simulink model "race"  (R2018a)
settings: Solver=VariableStepAuto  StartTime=0.0  StopTime=300  FixedStep=0.01  RelTol=1e-3
values from neighbouring files (symbols this model uses):
  gates = sim_gates(:,:,1)    [eval_sim.m]    (also in initialize_race_realtime.m = [dist,0,height,deg2rad(110); initialize_race_realtime_backup_cubic.m = [dist,0,height,deg2rad(110); plot_sim.m)
  splines = zeros(3,4,size(gates,1))    [initialize_race_no_realtime.m]    (also in show_splines.m)
undefined symbols (not defined in the file or in its folder): fspecial, gray, Rec, SDTV
libraries: visiontextngfix x2, visionanalysis x1, visiontransforms x1, visionconversions x1, vrlib x1
settings Model: Creator=vinni  LastModifiedBy=vinni

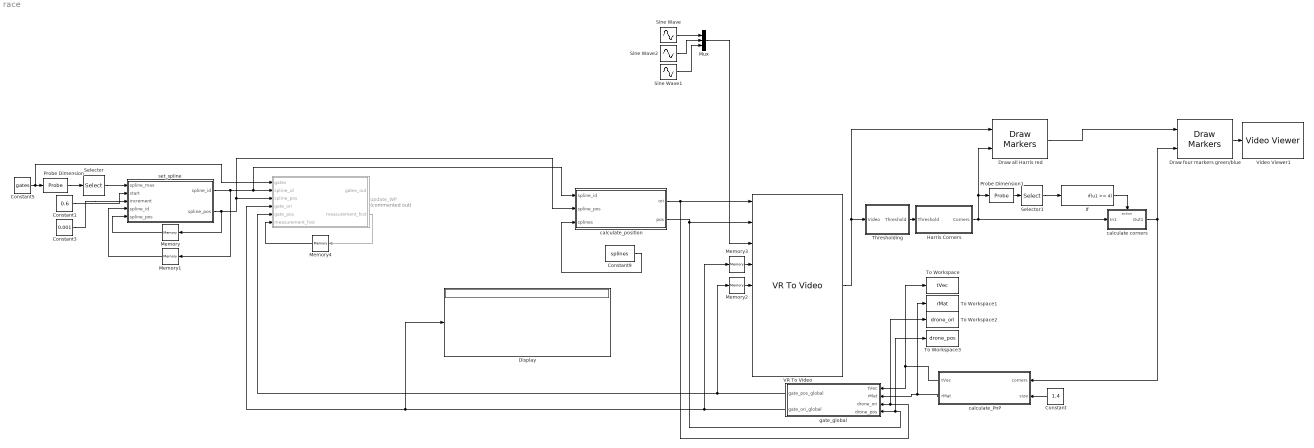
== system race ==
  Constant : Constant  Value=1.4
  Constant1 : Constant  Value=0.6
  Constant3 : Constant  Value=0.001
  Constant5 : Constant  Value=gates
  Constant9 : Constant  Value=splines
  Display : Display
  Draw all Harris red : visiontextngfix/Draw Markers  shape=Circle  size=3  fill=on  fillClrSource=Specify via dialog  display=User-specified value  intensity=200  color=[255 0 0]  opacity=1  viewport=Entire image  antialiasing=off  inType=Obsolete  imagePorts=One multidimensional signal  prodOutputMode=Binary point scaling  prodOutputWordLength=32  prodOutputFracLength=14  memoryMode=Specify word length  memoryWordLength=16  memoryFracLength=14  roundingMode=Floor  overflowMode=off
      settings: SourceProductName=Computer Vision System Toolbox  SourceProductBaseCode=VP
  Draw four markers green/blue : visiontextngfix/Draw Markers  shape=Circle  size=3  fill=on  fillClrSource=Specify via dialog  display=User-specified value  intensity=200  color=[0 255 0; 0 0 255;0 0 255; 0 255 0]  opacity=1  viewport=Entire image  antialiasing=off  inType=Obsolete  imagePorts=One multidimensional signal  prodOutputMode=Binary point scaling  prodOutputWordLength=32  prodOutputFracLength=14  memoryMode=Specify word length  memoryWordLength=16  memoryFracLength=14  roundingMode=Floor  overflowMode=off
      settings: SourceProductName=Computer Vision System Toolbox  SourceProductBaseCode=VP
  Harris Corners : Subsystem
  If : If  IfExpression=u1 >= 4  ShowElse=off
  Memory{,1..4} (5 alike) : Memory
  Mux : Mux  Inputs=3
  Probe Dimension : Probe  ProbeWidth=off  ProbeSampleTime=off  ProbeComplexSignal=off  ProbeSignalDimensions=on
  Probe Dimension1 : Probe  ProbeWidth=off  ProbeSampleTime=off  ProbeComplexSignal=off  ProbeSignalDimensions=on
  Selector : Selector  IndexOptions=Index vector (dialog)  Indices=1  OutputSizes=1
  Selector1 : Selector  IndexOptions=Index vector (dialog)  Indices=1  OutputSizes=1
  Sine Wave : Sin  Amplitude=0.0  Bias=3  Frequency=0.4  SampleTime=0
  Sine Wave1 : Sin  Amplitude=0.0  Bias=2  Frequency=0.4  SampleTime=0
  Sine Wave2 : Sin  Amplitude=0.0  Frequency=0.4  SampleTime=0
  Thresholding : Subsystem
  To Workspace : ToWorkspace  VariableName=tVec  SaveFormat=Timeseries  SampleTime=-1
  To Workspace1 : ToWorkspace  VariableName=rMat  SaveFormat=Timeseries  SampleTime=-1
  To Workspace2 : ToWorkspace  VariableName=drone_ori  SaveFormat=Timeseries  SampleTime=-1
  To Workspace3 : ToWorkspace  VariableName=drone_pos  SaveFormat=Timeseries  SampleTime=-1
  VR To Video : vrlib/VR To Video  InstantiateOnLoad=on  SampleTime=0.1  ViewEnable=on  RemoteChange=off  RemoteView=off  FieldsWritten=drone.orientation.4.1.1.double#drone.position.3.1.1.double#G1.translation.3.1.1.double#current_gate_red.rotation.4.1.1.double#current_gate_red.translation.3.1.1.double#current_gate_yellow.rotation.4.1.1.double#current_gate_yellow.translation.3.1.1.double#current_gate_green.rotation.4.1.1.double#current_gate_green.translation.3.1.1.double  WorldFileName=race_course.wrl  AutoView=off  VideoDimensions=1*[200 320]  AllowVariableSize=off  FigureProperties="{'Position', 'Name', 'Viewpoint', 'CameraBound', 'CameraDirection', 'CameraPosition', 'CameraUpVector', 'ZoomFactor', 'Antialiasing', 'Headlight', 'Lighting', 'NavPanel', 'Sound', 'StatusBar', 'Stereo3D', 'Stereo3DCameraOffset', 'Stereo3DHIT', 'ToolBar', 'Textures', 'Transparency', 'Triad', 'Wireframe', 'NavZones', 'NavMode', 'NavSpeed', 'CaptureFileFormat', 'CaptureFileName', 'Record2DCompressMethod', 'Record2DCompressQuality', 'Record2D', 'Record2DFileName', 'Record2DFPS'; [3.5500000000000000e+02   6.0000000000000000e+01   3.2000000000000000e+02   2.0000000000000000e+02], '', '_untitled_1', 'on', [0.0000000000000000e+00   0.0000000000000000e+00  -1.0000000000000000e+00], [0.0000000000000000e+00   0.0000000000000000e+00   0.0000000000000000e+00], [0.0000000000000000e+00   1.0000000000000000e+00   0.0000000000000000e+00], [1.0000000000000000e+00], 'on', 'on', 'on', 'none', 'on', 'off', 'off', [1.0000000149011612e-01], [0.0000000000000000e+00], 'off', 'on', 'on', 'none', 'off', 'off', 'fly', 'normal', 'tif', '%f_anim_%n.tif', 'auto', [7.5000000000000000e+01], 'off', '***video***', 'auto'}"
      settings: SourceProductName=Simulink 3D Animation  SourceProductBaseCode=VR
  Video Viewer1 : VideoViewer  colormapValue=gray(256)  FigPos=[66 898 1535 821]
  calculate corners : Subsystem  TreatAsAtomicUnit=on
  calculate_PnP : MATLAB Function  TreatAsAtomicUnit=on
  calculate_position : MATLAB Function  TreatAsAtomicUnit=on
  gate_global : MATLAB Function  TreatAsAtomicUnit=on
  set_spline : MATLAB Function  TreatAsAtomicUnit=on
  update_WP : MATLAB Function  Commented=on  TreatAsAtomicUnit=on
  wires:
  Sine Wave2/1 -> Mux/2
  Sine Wave/1 -> Mux/1
  Sine Wave1/1 -> Mux/3
  VR To Video/1 -> Draw all Harris red/1, Thresholding/1("Video ")
  Probe Dimension/1 -> Selector/1
  Selector/1 -> set_spline/1(spline_max)
  Constant5/1 -> update_WP/1(gates), Probe Dimension/1
  Memory1/1 -> set_spline/4("spline_id ")
  Memory/1 -> set_spline/5("spline_pos ")
  Constant9/1 -> calculate_position/3(splines)
  calculate_position/1(ori) -> To Workspace2/1, gate_global/3(drone_ori), VR To Video/1
  Draw all Harris red/1 -> Draw four markers green/blue/1
  Thresholding/1(Threshold) -> Harris Corners/1(Threshold)
  Harris Corners/1(Corners) -> Draw all Harris red/2, Probe Dimension1/1, calculate corners/1(In1)
  Constant/1 -> calculate_PnP/2(size)
  Probe Dimension1/1 -> Selector1/1
  Selector1/1 -> If/1
  calculate corners/1(Out1) -> calculate_PnP/1(corners), Draw four markers green/blue/2
  calculate_position/2(pos) -> To Workspace3/1, gate_global/4(drone_pos), VR To Video/2
  calculate_PnP/1(tVec) -> gate_global/1(tVec), To Workspace/1
  If/1 -> calculate corners/Action
  Draw four markers green/blue/1 -> Video Viewer1/1
  Constant3/1 -> set_spline/3(increment)
  calculate_PnP/2(rMat) -> gate_global/2(rMat), To Workspace1/1
  gate_global/1(gate_pos_global) -> update_WP/5(gate_pos), Memory2/1
  Constant1/1 -> set_spline/2(start)
  gate_global/2(gate_ori_global) -> Display/1, update_WP/4(gate_ori), Memory3/1
  Mux/1 -> VR To Video/3
  Memory3/1 -> VR To Video/4
  Memory2/1 -> VR To Video/5
  update_WP/2(measurement_hist) -> Memory4/1
  Memory4/1 -> update_WP/6("measurement_hist ")
  set_spline/1(spline_id) -> Memory1/1, calculate_position/1(spline_id), update_WP/2(spline_id)
  set_spline/2(spline_pos) -> Memory/1, calculate_position/2(spline_pos), update_WP/3(spline_pos)

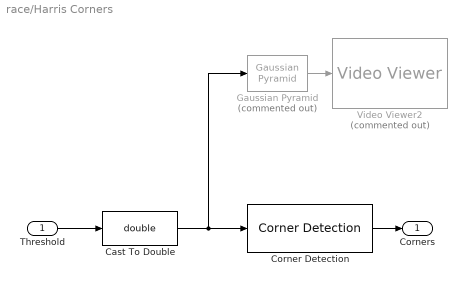
== system race/Harris Corners ==
  Threshold : Inport
  Cast To Double : DataTypeConversion  OutDataTypeStr=double
  Corner Detection : visionanalysis/Corner Detection  method=Harris corner detection (Harris & Stephens)  factor=0.01  filter=fspecial('gaussian', [1 9], 3)  thrInten=0.1  thrAngle=157.5  output=Obsolete9b  outputInUse=Corner location  maxNum=5  thrMetric=0.01  neighborSize=[25 25]  isOutVarDim=on  accumMode=Binary point scaling  accumWordLength=32  accumFracLength=0  prodOutputMode=Binary point scaling  prodOutputWordLength=32  prodOutputFracLength=0  memoryMode=Binary point scaling  memoryWordLength=32  memoryFracLength=0  firstCoeffMode=Specify word length  firstCoeffWordLength=16  firstCoeffFracLength=17  roundingMode=Floor  overflowMode=off
      settings: SourceProductName=Computer Vision System Toolbox  SourceProductBaseCode=VP
  Gaussian Pyramid : visiontransforms/Gaussian Pyramid  Commented=on  operation=Expand  level=1  source=Specify via dialog  a=0.375  coef=fspecial('gaussian', [1 9], 3)  hiddenCoef=fspecial('gaussian', [1 9], 3)  firstCoeffMode=Specify word length  firstCoeffWordLength=16  firstCoeffFracLength=17  outputMode=Binary point scaling  outputWordLength=32  outputFracLength=10  prodOutputMode=Binary point scaling  prodOutputWordLength=32  prodOutputFracLength=10  roundingMode=Floor  overflowMode=off
      settings: SourceProductName=Computer Vision System Toolbox  SourceProductBaseCode=VP
  Video Viewer2 : VideoViewer  Commented=on  colormapValue=gray(256)  FigPos=[66 898 768 793]
  Corners : Outport
  wires:
  Threshold/1 -> Cast To Double/1
  Cast To Double/1 -> Gaussian Pyramid/1, Corner Detection/1
  Gaussian Pyramid/1 -> Video Viewer2/1
  Corner Detection/1 -> Corners/1

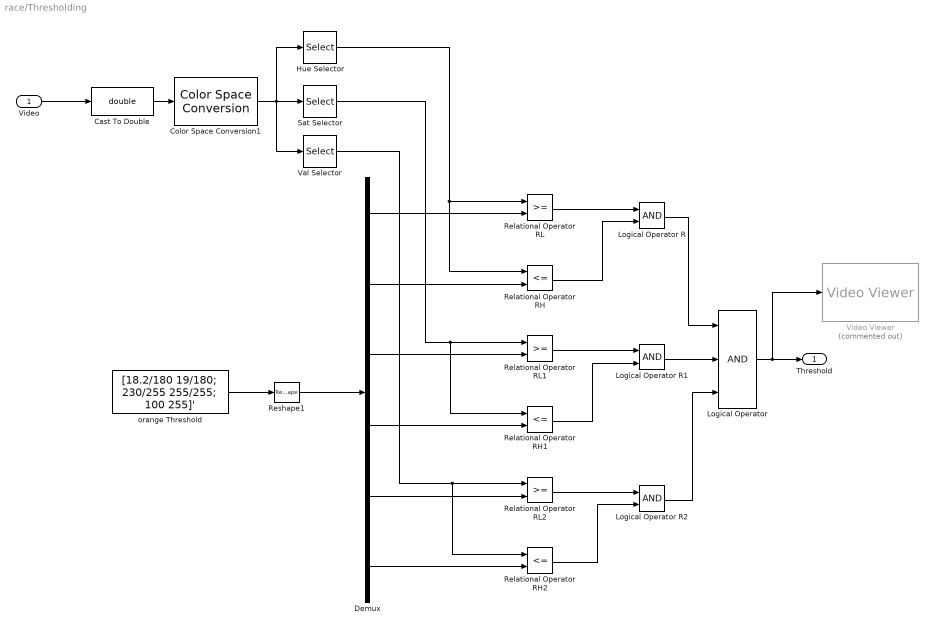
== system race/Thresholding ==
  "Video " : Inport
  Cast To Double : DataTypeConversion  OutDataTypeStr=double
  Color Space Conversion1 : visionconversions/Color Space  Conversion  conversion=Obsolete  conversionActive=R'G'B' to HSV  wp_str=D65  rec=Rec. 601 (SDTV)  sys=1125/60/2:1  imagePorts=One multidimensional signal
      settings: SourceProductName=Computer Vision System Toolbox
  Demux : Demux  Outputs=6
  Hue Selector : Selector  NumberOfDimensions=3  InputPortWidth=3  IndexOptions=Select all,Select all,Index vector (dialog)  Indices=[1 3],1,1  OutputSizes=1,1,1
  Logical Operator : Logic  Inputs=3  AllPortsSameDT=off  OutDataTypeStr=boolean
  Logical Operator R : Logic  AllPortsSameDT=off  OutDataTypeStr=boolean
  Logical Operator R1 : Logic  AllPortsSameDT=off  OutDataTypeStr=boolean
  Logical Operator R2 : Logic  AllPortsSameDT=off  OutDataTypeStr=boolean
  Relational Operator RH : RelationalOperator  Operator=<=  OutDataTypeStr=boolean  RndMeth=Nearest
  Relational Operator RH1 : RelationalOperator  Operator=<=  OutDataTypeStr=boolean  RndMeth=Nearest
  Relational Operator RH2 : RelationalOperator  Operator=<=  OutDataTypeStr=boolean  RndMeth=Nearest
  Relational Operator RL : RelationalOperator  OutDataTypeStr=boolean  RndMeth=Nearest
  Relational Operator RL1 : RelationalOperator  OutDataTypeStr=boolean  RndMeth=Nearest
  Relational Operator RL2 : RelationalOperator  OutDataTypeStr=boolean  RndMeth=Nearest
  Reshape1 : Reshape
  Sat Selector : Selector  NumberOfDimensions=3  InputPortWidth=3  IndexOptions=Select all,Select all,Index vector (dialog)  Indices=[1 3],1,2  OutputSizes=1,1,1
  Val Selector : Selector  NumberOfDimensions=3  InputPortWidth=3  IndexOptions=Select all,Select all,Index vector (dialog)  Indices=[1 3],1,3  OutputSizes=1,1,1
  Video Viewer : VideoViewer  Commented=on  colormapValue=gray(256)  FigPos=[66 898 1535 821]
  orange Threshold : Constant  Value=[18.2/180 19/180; 230/255 255/255; 100 255]'  OutDataTypeStr=double
  Threshold : Outport
  wires:
  Color Space Conversion1/1 -> Val Selector/1, Sat Selector/1, Hue Selector/1
  Demux/6 -> Relational Operator RH2/2
  Val Selector/1 -> Relational Operator RH2/1, Relational Operator RL2/1
  Demux/3 -> Relational Operator RL1/2
  Relational Operator RL/1 -> Logical Operator R/1
  Demux/2 -> Relational Operator RH/2
  orange Threshold/1 -> Reshape1/1
  Cast To Double/1 -> Color Space Conversion1/1
  Demux/5 -> Relational Operator RL2/2
  Hue Selector/1 -> Relational Operator RH/1, Relational Operator RL/1
  Logical Operator R/1 -> Logical Operator/1
  Relational Operator RH/1 -> Logical Operator R/2
  Demux/1 -> Relational Operator RL/2
  Demux/4 -> Relational Operator RH1/2
  "Video "/1 -> Cast To Double/1
  Reshape1/1 -> Demux/1
  Logical Operator R1/1 -> Logical Operator/2
  Relational Operator RH1/1 -> Logical Operator R1/2
  Sat Selector/1 -> Relational Operator RH1/1, Relational Operator RL1/1
  Relational Operator RL1/1 -> Logical Operator R1/1
  Relational Operator RH2/1 -> Logical Operator R2/2
  Relational Operator RL2/1 -> Logical Operator R2/1
  Logical Operator R2/1 -> Logical Operator/3
  Logical Operator/1 -> Video Viewer/1, Threshold/1

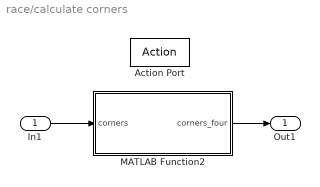
== system race/calculate corners ==
  In1 : Inport
  Action Port : ActionPort  PropagateVarSize=During execution  ActionType=then
  MATLAB Function2 : MATLAB Function  TreatAsAtomicUnit=on
  Out1 : Outport
  wires:
  In1/1 -> MATLAB Function2/1(corners)
  MATLAB Function2/1(corners_four) -> Out1/1

== matlab function race/calculate_position ==
  data: spline_id input; spline_pos input; ori output; splines input; pos output
function [ori, pos] = calculate_position(spline_id,spline_pos,splines)
    
    spline_para = splines(:,:,spline_id);
    P0 = spline_para(1,:);
    P1 = spline_para(2,:);
    P2 = spline_para(3,:);
    
    unit=ones(1,size(P0,2));
    d = spline_pos;
    pos_t = (1-d)*unit.*((1-d)*P0+d*P1)+d*unit.*((1-d)*P1 + d*P2);
    pos = pos_t(1:3)';
    hdg = pos_t(4);
    
    sRg = eul2rotm([-pi/2, 0, pi/2]);
    gRd = eul2rotm([0, hdg, 0]);
    
    sRd = sRg*gRd;
    ori_t = rotm2axang(sRd); 
    ori = ori_t';
    
end

== matlab function race/set_spline ==
  data: spline_max input; start input; increment input; spline_id output; spline_id input; spline_pos input; spline_pos output
function [spline_id,spline_pos] = set_spline(spline_max,start,increment,spline_id,spline_pos)
    
    if spline_id == 0
        spline_id = 1;
        spline_pos = start;
    else
        spline_pos = spline_pos + increment;
    end
    
    if spline_pos > 1
        spline_pos = spline_pos - 1;
        spline_id = spline_id + 1;
    end

    if spline_id > spline_max
        spline_id = 1;
    end

end

== matlab function race/calculate corners/MATLAB Function2 ==
  data: corners_four output; corners input
function corners_four = calculate_corners(corners)
    
    
    %% get bounding box
    corners = double(corners);
    box=[0,0,0,0];
    box(1) = min(corners(:,1));
    box(2) = max(corners(:,1));
    box(3) = min(corners(:,2));
    box(4) = max(corners(:,2));
    
    corners_box = ([box(1), box(3);
                    box(2), box(3);
                    box(1), box(4);
                    box(2), box(4)]);
                
    corners_four = int32(zeros(4,2));
                
    for m = 1:4
        box = corners_box(m,:);
        multi_box = ones(size(corners,1),1) * box;
        diff = multi_box - corners;
        dist = diff(:,1).^2 + diff(:,2).^2;
        [~,i] = min(dist);
        corners_four(m,:) = corners(i,:);
        corners(i,:)=[];
    end
    
end

== matlab function race/calculate_PnP ==
  data: tVec output; rMat output; corners input; size input
function [tVec, rMat] = calculate_PnP(corners, size)
    tVec=zeros(1,3);
    rMat=zeros(3,3);
    
    Resolution = 1*[320, 200];
    vertFOV = 1.05;
    f = 0.5*Resolution(2)/tan(0.5*vertFOV);
    IntrinsicMatrix = [f, 0, 0;
        0, f, 0;
        Resolution/2, 1];
    cameraParams = cameraParameters('IntrinsicMatrix',IntrinsicMatrix); 
    
    %% calculate extrinsics
    worldPoints = size/2*[1 1;
        1 -1;
        -1 1;
        -1 -1];
    
    corners=double(corners);
    
    angles = zeros(6,1);
    k = 1;
    for m=1:3
        for n=m+1:4
            angles(k)=atan2(corners(m,2)-corners(n,2),corners(m,1)-corners(n,1));
            k = k+1;            
        end
    end
    angles(angles<=0) = angles(angles<=0)+pi;
    
    a = hist(angles,unique(angles));
    if max(a)>2
        disp('three occurences')
        return
    end
    
    
    
    angles = zeros(2,1);
    angles(1)=atan2(corners(1,2)-corners(4,2),corners(1,1)-corners(4,1));
    angles(2)=atan2(corners(2,2)-corners(3,2),corners(2,1)-corners(3,1));
    angles(angles<=0) = angles(angles<=0)+pi;
    
    if ~(isequal(unique(angles),sort(angles)))
        temp = corners(3,:);
        corners(3,:) = corners(4,:);
        corners(4,:) = temp;
    end
    
    angles(1)=atan2(corners(1,2)-corners(4,2),corners(1,1)-corners(4,1));
    angles(2)=atan2(corners(2,2)-corners(3,2),corners(2,1)-corners(3,1));
    angles(angles<=0) = angles(angles<=0)+pi;
    
    if ~(isequal(unique(angles),sort(angles)))
        corners
        disp('still bad after sort')
        return
    end    
    
    [rMat,tVec] = extrinsics(corners,worldPoints,cameraParams);
%     [orientation,location] = extrinsicsToCameraPose(rMat,tVec);
    
end

== matlab function race/gate_global ==
  data: gate_pos_global output; tVec input; rMat input; drone_ori input; drone_pos input; gate_ori_global output
function [gate_pos_global, gate_ori_global]  = gate_global(tVec, rMat, drone_ori, drone_pos)

    gate_pos_global = zeros(3,1);
    gate_ori_global = zeros(4,1);
%     drone_rotm = axang2rotm(drone_ori');
%     gate_pos_local = quatrotate(drone_q,gate_pos_cam);
%     gate_pos_local = drone_rotm * gate_pos_cam';
%     gate_pos_global = gate_pos_local + drone_pos';
%     gate_pos_global = gate_pos_local;
    
    
    %% drone pos
    drone_pos;
    
    
    %% drone orientation
    dRs = axang2rotm(drone_ori');
    gRs = eul2rotm([-pi/2, 0, pi/2]);
    sRg = gRs^-1;
    dRg = dRs*sRg;
    
    
    %% convert gate pos
    % tVec = right down front, drone was front left up
    dRc = eul2rotm([pi/2,-pi/2,0],'ZYX');
    cRd = dRc^-1;
    cRg = dRg*cRd;
    rel= cRg*tVec';
    gate_pos_global = drone_pos + rel;
    
    % rel = -dRs*tvec';
    % gate_pos_global = drone_pos + rel';
    
    
    %% convert gate orientation
    wRc = rMat;
    one_more = eul2rotm([-pi/2,pi/2,0]);
    another_one = 1;%eul2rotm([0,-pi/2,0]);
    wRs = another_one*one_more*wRc*cRg^-1;
    
    gate_ori_global = (rotm2axang(wRs))';

    
end

== matlab function race/update_WP ==
  data: gates_out output; gates input; spline_id input; spline_pos input; gate_ori input; gate_pos input; measurement_hist input; measurement_hist output
function [gates_out, measurement_hist]   = update_WP(gates, spline_id, spline_pos, gate_ori, gate_pos, measurement_hist)

    %% setup history
    if measurement_hist == 0 || (spline_pos > 0.95 && ~(measurement_hist == ones(5,1)*gates(1,:)))
        measurement_hist = ones(5,1)*gates(1,:);
    end
    
    %% calculate average
    average_pos = mean(measurement_hist(:,1:3));
    hdgs = unwrap(measurement_hist(:,4));
    average_hdg = atan2(sum(sin(hdgs)),sum(cos(hdgs)));
    
    %% verify measurement
    
    
    %% calculate new average and set as gate
    gates_out = gates;
    
end
